simulink model "dampmaskine_rev9"  (R2017b)
settings: Solver=ode45  StartTime=0.0  StopTime=1000  RelTol=2e-6  EnableMultiTasking=on
values from neighbouring files (symbols this model uses):
  Bm = 2e-6    (= 2e-06)    [konstanter_rev9.m]
  CthV1 = 5    [konstanter_rev9.m]
  CthV2 = 50    [konstanter_rev9.m]
  Jm = Jmm + 0.5 * (0.015^2 * pi * 0.03 * jernMassefylde) * 0.015^2    (= 0.000106908078188)    [konstanter_rev9.m]
  Kd = stempelAreal*krumtapArm/2 * kd_ny * antalCylindre    (= 1.01787601976e-07)    [konstanter_rev9.m]
  kedelGodsVarmekapacitet = kedelOverflade*kedelGodsTykkelse * jernMassefylde * jernVarmefylde    (= 211.895159678)    [konstanter_rev9.m]
  kedelOverflade = 2 * (kedelDiameter / 2)^2 * pi + kedelDiameter * pi * kedelLength    (= 0.0403757487839)    [konstanter_rev9.m]
  kedelVandVarmekapacitet = kedelVolumen * vandMassefylde * vandVarmefylde    (= 2110.84160173)    [konstanter_rev9.m]
  kedelVolumen = (kedelDiameter / 2 - kedelGodsTykkelse)^2 * pi * (kedelLength - kedelGodsTykkelse*2)    (= 0.000504382700534)    [konstanter_rev9.m]
  Kp = 1/M    [Opgave33.m]    (also in konstanter_rev9.m = 3360.3; tfAfDamp_konstanter.m)
  Kvm = 1/(1-spild)*stempelAreal * slaglng / (2 * pi) * fyndningsgrad * antalCylindre    (= 9.25714285714e-07)    [konstanter_rev9.m]
  polPrRad = 13/(2*pi)    (= 2.06901426019)    [konstanter_rev9.m]
  RthV1 = 0.3    [konstanter_rev9.m]
  RthV2 = 0.1    [konstanter_rev9.m]
  startFriction = 0.005    [konstanter_rev9.m]
  tau_i = Ni/omega_c    (= 0.46511627907)    [Opgave33.m]    (also in konstanter_rev9.m = 32.05; tfAfDamp_konstanter.m = 32.0512820513)
  voltPerRad = voltPerRPM*60/2/pi    (= 0.019098593171)    [konstanter_rev9.m]
settings Model: Creator=chr  LastModifiedBy=tilfr
settings SolverCC: ZeroCrossAlgorithm=Adaptive
settings DataIOCC: MaxDataPoints=2000  SaveFinalState=on  SaveFormat=Array
settings OptimizationCC: ExpressionDepthLimit=2147483647  LifeSpan=inf
settings DebuggingCC: UnderspecifiedInitializationDetection=Classic  MergeDetectMultiDrivingBlocksExec=none  SolverPrmCheckMsg=warning  MultiTaskDSMMsg=warning  MultiTaskCondExecSysMsg=none  FcnCallInpInsideContextMsg=warning  StateNameClashWarn=warning  SFUnexpectedBacktrackingDiag=warning  SFNoUnconditionalDefaultTransitionDiag=warning  SFExecutionAtInitializationDiag=none
settings HardwareCC: ProdBitPerPointer=32  ProdBitPerSizeT=32  ProdBitPerPtrDiffT=32  ProdLargestAtomicFloat=None  ProdIntDivRoundTo=Undefined  ProdEndianess=Unspecified  ProdWordSize=32  ProdHWDeviceType=32-bit Generic
settings ModelReferenceCC: PropagateSignalLabelsOutOfModel=off
settings CodeAppCC: StateflowObjectComments=on
settings GRTTargetCC: TargetLangStandard=C89/C90 (ANSI)  GeneratePreprocessorConditionals=Disable all
settings ConfigComp: CovMetricSettings=dw  CovHtmlReporting=on  CovSaveCumulativeToWorkspaceVar=on  CovSaveSingleToWorkspaceVar=on  CovExternalEMLEnable=off
settings ConfigurationSet: Description=SimMechanics 2G

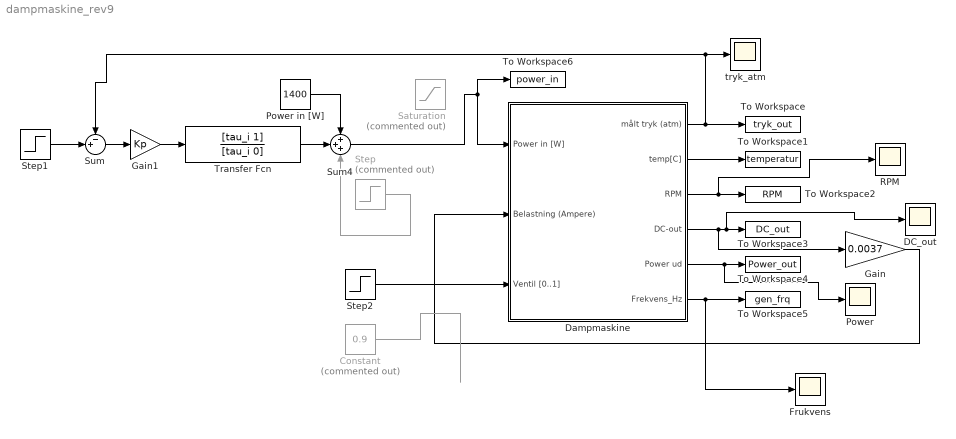
== system dampmaskine_rev9 ==
  Constant : Constant  Commented=on  Value=0.9
  DC_out : Scope
  Dampmaskine : Subsystem
  Frukvens : Scope
  Gain : Gain  Gain=0.0037
  Gain1 : Gain  Gain=Kp
  Power : Scope
  Power in [W] : Constant  Value=1400
  RPM : Scope
  Saturation : Saturate  Commented=on  UpperLimit=1400  LowerLimit=0
  Step : Step  Commented=on  Time=150  After=-50  SampleTime=0
  Step1 : Step  Time=0  After=3  SampleTime=0
  Step2 : Step  Time=500  Before=0.5  After=0.6  SampleTime=0
  Sum : Sum  Inputs=-+|
  Sum4 : Sum  Inputs=+++
  To Workspace : ToWorkspace  VariableName=tryk_out  SaveFormat=Timeseries  SampleTime=0.1
  To Workspace1 : ToWorkspace  VariableName=temperatur  SaveFormat=Timeseries  SampleTime=-1
  To Workspace2 : ToWorkspace  VariableName=RPM  SaveFormat=Timeseries  SampleTime=-1
  To Workspace3 : ToWorkspace  VariableName=DC_out  SaveFormat=Timeseries  SampleTime=-1
  To Workspace4 : ToWorkspace  VariableName=Power_out  SaveFormat=Timeseries  SampleTime=-1
  To Workspace5 : ToWorkspace  VariableName=gen_frq  SaveFormat=Timeseries  SampleTime=0.1
  To Workspace6 : ToWorkspace  VariableName=power_in  SaveFormat=Timeseries  SampleTime=0.1
  Transfer Fcn : TransferFcn  Numerator=[tau_i 1]  Denominator=[tau_i 0]
  tryk_atm : Scope
  wires:
  Step2/1 -> Dampmaskine/3(Ventil [0..1])
  Dampmaskine/3(RPM) -> RPM/1, To Workspace2/1
  Dampmaskine/6(Frekvens_Hz) -> Frukvens/1, To Workspace5/1
  Dampmaskine/5(Power ud) -> Power/1, To Workspace4/1
  Dampmaskine/2(temp[C]) -> To Workspace1/1
  Dampmaskine/4(DC-out) -> Gain/1, DC_out/1, To Workspace3/1
  Dampmaskine/1(målt tryk (atm)) -> Sum/1, tryk_atm/1, To Workspace/1
  Power in [W]/1 -> Sum4/1
  Step/1 -> Sum4/3
  Gain/1 -> Dampmaskine/2(Belastning (Ampere))
  Sum4/1 -> Dampmaskine/1(Power in [W]), To Workspace6/1
  Transfer Fcn/1 -> Sum4/2
  Gain1/1 -> Transfer Fcn/1
  Step1/1 -> Sum/2
  Sum/1 -> Gain1/1
  Constant/1 -> ?

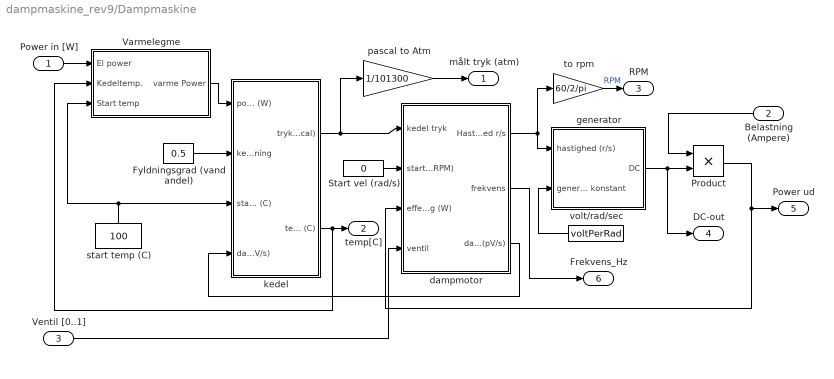
== system dampmaskine_rev9/Dampmaskine ==
  Power in [W] : Inport
  Belastning (Ampere) : Inport  Port=2
  Ventil [0..1] : Inport  Port=3
  Fyldningsgrad (vand andel) : Constant  Value=0.5
  Product : Product  RndMeth=Zero
  Start vel (rad/s) : Constant  Value=0
  Varmelegme : Subsystem
  dampmotor : Subsystem
  generator : Subsystem
  kedel : Subsystem
  pascal to Atm : Gain  Gain=1/101300
  start temp (C) : Constant  Value=100
  to rpm : Gain  Gain=60/2/pi
  volt/rad/sec : Constant  Value=voltPerRad
  målt tryk (atm) : Outport
  temp[C] : Outport  Port=2
  RPM : Outport  Port=3
  DC-out : Outport  Port=4
  Power ud : Outport  Port=5
  Frekvens_Hz : Outport  Port=6
  wires:
  Fyldningsgrad (vand andel)/1 -> kedel/2(kedel fyldning)
  start temp (C)/1 -> Varmelegme/3(Start temp), kedel/3(start temp (C))
  dampmotor/1(Hastighed r/s) -> generator/1(hastighed (r/s)), to rpm/1
  volt/rad/sec/1 -> generator/2(generator konstant)
  pascal to Atm/1 -> målt tryk (atm)/1
  Start vel (rad/s)/1 -> dampmotor/2(start vel (RPM))
  kedel/1(tryk (pascal)) -> pascal to Atm/1, dampmotor/1(kedel tryk)
  to rpm/1 -> RPM/1  "RPM"
  kedel/2(temp (C)) -> Varmelegme/2(Kedeltemp.), temp[C]/1
  dampmotor/3(damp forbrug (pV/s)) -> kedel/4(dampflow (pV/s))
  Belastning (Ampere)/1 -> Product/1
  generator/1(DC) -> Product/2, DC-out/1
  Product/1 -> dampmotor/3(effekt forbrug (W)), Power ud/1
  Power in [W]/1 -> Varmelegme/1(El power)
  Varmelegme/1(varme Power) -> kedel/1(power ind  (W))
  Ventil [0..1]/1 -> dampmotor/4(ventil)
  dampmotor/2(frekvens) -> Frekvens_Hz/1

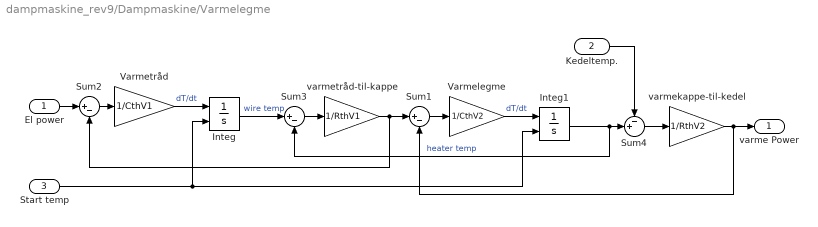
== system dampmaskine_rev9/Dampmaskine/Varmelegme ==
  El power : Inport
  Kedeltemp. : Inport  Port=2
  Start temp : Inport  Port=3
  Integ : Integrator  InitialConditionSource=external
  Integ1 : Integrator  InitialConditionSource=external
  Sum1 : Sum  Inputs=|+-
  Sum2 : Sum  Inputs=|+-
  Sum3 : Sum  Inputs=|+-
  Sum4 : Sum  Inputs=-+|
  Varmelegme : Gain  Gain=1/CthV2
  Varmetråd : Gain  Gain=1/CthV1
  varmekappe-til-kedel : Gain  Gain=1/RthV2
  varmetråd-til-kappe : Gain  Gain=1/RthV1
  varme Power : Outport
  wires:
  Sum3/1 -> varmetråd-til-kappe/1
  El power/1 -> Sum2/1
  Varmetråd/1 -> Integ/1  "dT/dt"
  Sum2/1 -> Varmetråd/1
  Integ/1 -> Sum3/1  "wire temp"
  Sum4/1 -> varmekappe-til-kedel/1
  Kedeltemp./1 -> Sum4/1
  varmetråd-til-kappe/1 -> Sum1/1, Sum2/2
  Varmelegme/1 -> Integ1/1  "dT/dt"
  Sum1/1 -> Varmelegme/1
  Integ1/1 -> Sum4/2, Sum3/2  "heater temp"
  varmekappe-til-kedel/1 -> varme Power/1, Sum1/2
  Start temp/1 -> Integ1/2, Integ/2

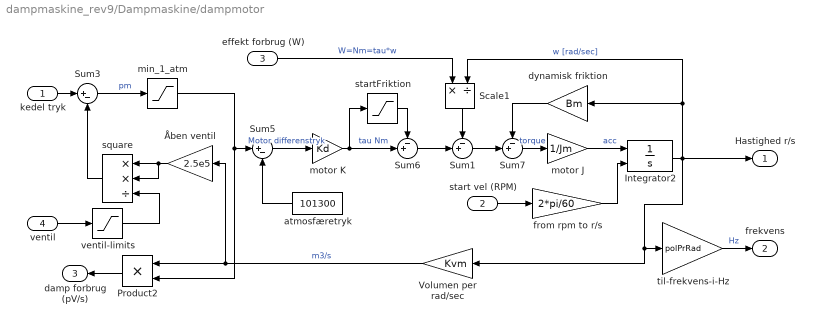
== system dampmaskine_rev9/Dampmaskine/dampmotor ==
  kedel tryk : Inport
  start vel (RPM) : Inport  Port=2
  effekt forbrug (W) : Inport  Port=3
  ventil : Inport  Port=4
  Integrator2 : Integrator  InitialConditionSource=external  InitialCondition=1332/60*2*pi  LimitOutput=on  LowerSaturationLimit=0.001
  Product2 : Product  RndMeth=Zero
  Scale1 : Product  Inputs=*/
  Sum1 : Sum  Inputs=-+|
  Sum3 : Sum  Inputs=|+-
  Sum5 : Sum  Inputs=|+-
  Sum6 : Sum  Inputs=-+|
  Sum7 : Sum  Inputs=-+|
  Volumen per rad/sec : Gain  Gain=Kvm
  atmosfæretryk : Constant  Value=101300
  dynamisk friktion : Gain  Gain=Bm
  from rpm to r/s : Gain  Gain=2*pi/60
  min_1_atm : Saturate  UpperLimit=1e8  LowerLimit=101300
  motor J : Gain  Gain=1/Jm
  motor K : Gain  Gain=Kd
  square : Product  Inputs=**/  RndMeth=Zero
  startFriktion : Saturate  UpperLimit=startFriction  LowerLimit=-startFriction
  til-frekvens-i-Hz : Gain  Gain=polPrRad
  ventil-limits : Saturate  UpperLimit=1  LowerLimit=1e-5
  Åben ventil : Gain  Gain=2.5e5
  Hastighed r/s : Outport
  frekvens : Outport  Port=2
  damp forbrug (pV/s) : Outport  Port=3
  wires:
  Sum5/1 -> motor K/1  "Motor differenstryk"
  atmosfæretryk/1 -> Sum5/2
  Sum7/1 -> motor J/1  "torque"
  motor J/1 -> Integrator2/1  "acc"
  Integrator2/1 -> Hastighed r/s/1, Scale1/2, dynamisk friktion/1, Volumen per rad/sec/1, til-frekvens-i-Hz/1  "w [rad/sec]"
  dynamisk friktion/1 -> Sum7/1
  motor K/1 -> startFriktion/1, Sum6/2  "tau Nm"
  Sum3/1 -> min_1_atm/1  "pm"
  Åben ventil/1 -> square/2, square/1
  Volumen per rad/sec/1 -> Åben ventil/1, Product2/1  "m3/s"
  min_1_atm/1 -> Product2/2, Sum5/1
  kedel tryk/1 -> Sum3/1
  Product2/1 -> damp forbrug (pV/s)/1
  effekt forbrug (W)/1 -> Scale1/1  "W=Nm=tau*w"
  square/1 -> Sum3/2
  start vel (RPM)/1 -> from rpm to r/s/1
  from rpm to r/s/1 -> Integrator2/2
  ventil/1 -> ventil-limits/1
  ventil-limits/1 -> square/3
  til-frekvens-i-Hz/1 -> frekvens/1  "Hz"
  Sum1/1 -> Sum7/2
  Sum6/1 -> Sum1/2
  Scale1/1 -> Sum1/1
  startFriktion/1 -> Sum6/1

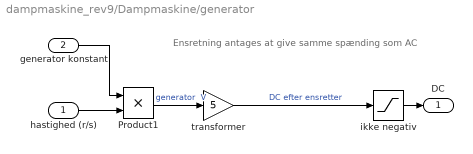
== system dampmaskine_rev9/Dampmaskine/generator ==
  note: Ensretning antages at give samme spænding som AC
  hastighed (r/s) : Inport
  generator konstant : Inport  Port=2
  Product1 : Product  RndMeth=Zero
  ikke negativ : Saturate  UpperLimit=300  LowerLimit=0
  transformer : Gain  Gain=5
  DC : Outport
  wires:
  hastighed (r/s)/1 -> Product1/2
  Product1/1 -> transformer/1  "generator  V"
  generator konstant/1 -> Product1/1
  transformer/1 -> ikke negativ/1  "DC efter ensretter"
  ikke negativ/1 -> DC/1

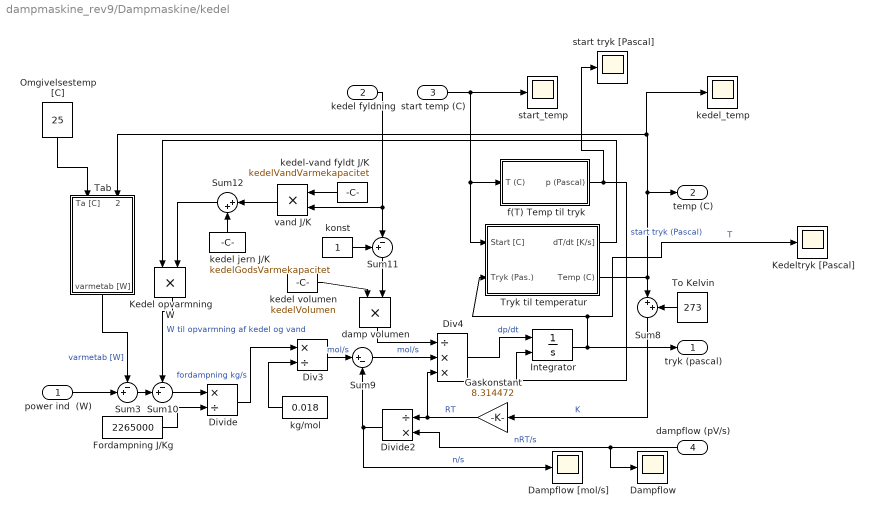
== system dampmaskine_rev9/Dampmaskine/kedel ==
  power ind  (W) : Inport
  kedel fyldning : Inport  Port=2
  start temp (C) : Inport  Port=3
  dampflow (pV/s) : Inport  Port=4
  Dampflow : Scope
  Dampflow [mol/s] : Scope
  Div3 : Product  Inputs=*/
  Div4 : Product  Inputs=/**
  Divide : Product  Inputs=*/
  Divide2 : Product  Inputs=/*
  Fordampning J/Kg : Constant  Value=2265000
  Gaskonstant : Gain  Gain=8.314472
  Integrator : Integrator  InitialConditionSource=external  InitialCondition=122.7
  Kedel opvarmning W : Product  RndMeth=Zero
  Kedeltryk [Pascal] : Scope
  Omgivelsestemp [C] : Constant  Value=25
  Sum10 : Sum  Inputs=-+|
  Sum11 : Sum  Inputs=+-|
  Sum12 : Sum  Inputs=|++
  Sum3 : Sum  Inputs=-+|
  Sum8 : Sum  Inputs=|++
  Sum9 : Sum  Inputs=|+-
  Tab : Subsystem
  To Kelvin : Constant  Value=273
  Tryk til temperatur : Subsystem
  damp volumen : Product  RndMeth=Zero
  f(T) Temp til tryk : Subsystem
  kedel jern J/K : Constant  Value=kedelGodsVarmekapacitet
  "kedel volumen " : Constant  Value=kedelVolumen
  kedel-vand fyldt J/K : Constant  Value=kedelVandVarmekapacitet
  kedel_temp : Scope
  kg/mol : Constant  Value=0.018
  konst : Constant
  start tryk [Pascal] : Scope
  "start_temp " : Scope
  vand J/K : Product  RndMeth=Zero
  tryk (pascal) : Outport
  temp (C) : Outport  Port=2
  wires:
  f(T) Temp til tryk/1(p (Pascal)) -> start tryk [Pascal]/1, Integrator/2  "start tryk (Pascal)"
  Gaskonstant/1 -> Div4/3, Divide2/1  "RT"
  Divide2/1 -> Dampflow [mol/s]/1, Sum9/2  "n/s"
  dampflow (pV/s)/1 -> Dampflow/1, Divide2/2  "nRT/s"
  Fordampning J/Kg/1 -> Divide/2
  Divide/1 -> Div3/1  "fordampning kg/s"
  kg/mol/1 -> Div3/2
  Div3/1 -> Sum9/1  "mol/s"
  Integrator/1 -> tryk (pascal)/1, Kedeltryk [Pascal]/1, Tryk til temperatur/2(Tryk (Pas.))  "T"
  Div4/1 -> Integrator/1  "dp/dt"
  To Kelvin/1 -> Sum8/2
  Sum8/1 -> Gaskonstant/1  "K"
  Sum3/1 -> Sum10/2
  Kedel opvarmning W/1 -> Sum10/1  "W til opvarmning af kedel og vand"
  Sum10/1 -> Divide/1
  Sum9/1 -> Div4/2  "mol/s"
  damp volumen/1 -> Div4/1
  "kedel volumen "/1 -> damp volumen/1
  Sum11/1 -> damp volumen/2
  kedel fyldning/1 -> Sum11/2, vand J/K/2
  kedel-vand fyldt J/K/1 -> vand J/K/1
  vand J/K/1 -> Sum12/1
  Sum12/1 -> Kedel opvarmning W/2
  kedel jern J/K/1 -> Sum12/2
  konst/1 -> Sum11/1
  start temp (C)/1 -> Tryk til temperatur/1(Start [C]), f(T) Temp til tryk/1(T (C)), "start_temp "/1
  Tryk til temperatur/2(Temp (C)) -> kedel_temp/1, Tab/2(Kedel temp), temp (C)/1, Sum8/1
  Tryk til temperatur/1(" dT/dt [K/s]") -> Kedel opvarmning W/1
  Tab/1(varmetab [W]) -> Sum3/1  "varmetab [W]"
  Omgivelsestemp [C]/1 -> Tab/1(Ta [C])
  power ind  (W)/1 -> Sum3/2

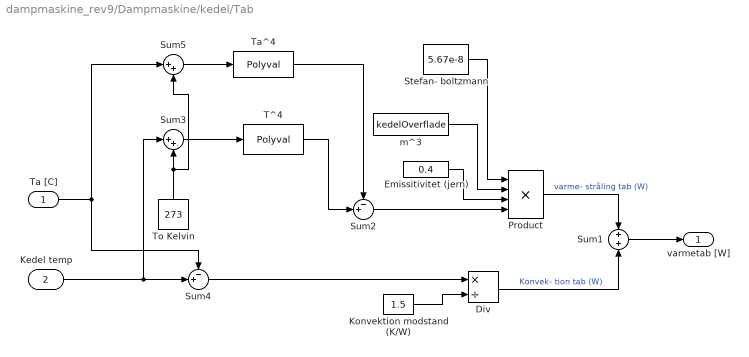
== system dampmaskine_rev9/Dampmaskine/kedel/Tab ==
  Ta [C] : Inport
  Kedel temp : Inport  Port=2
  Div : Product  Inputs=*/
  Emissitivitet (jern) : Constant  Value=0.4
  Konvektion modstand (K/W) : Constant  Value=1.5
  Product : Product  Inputs=4  RndMeth=Zero
  Stefan- boltzmann : Constant  Value=5.67e-8
  Sum1 : Sum  Inputs=+|+
  Sum2 : Sum  Inputs=-+|
  Sum3 : Sum  Inputs=|++
  Sum4 : Sum  Inputs=-+|
  Sum5 : Sum  Inputs=|++
  T^4 : Polyval  Coefs=[1,0,0,0,0 ]
  Ta^4 : Polyval  Coefs=[1,0,0,0,0 ]
  To Kelvin : Constant  Value=273
  m^3 : Constant  Value=kedelOverflade
  varmetab [W] : Outport
  wires:
  Ta^4/1 -> Sum2/1
  Kedel temp/1 -> Sum3/1, Sum4/2
  Sum2/1 -> Product/4
  Ta [C]/1 -> Sum4/1, Sum5/1
  Stefan- boltzmann/1 -> Product/1
  Emissitivitet (jern)/1 -> Product/3
  Sum3/1 -> T^4/1
  T^4/1 -> Sum2/2
  Sum4/1 -> Div/1
  Sum5/1 -> Ta^4/1
  Div/1 -> Sum1/2  "Konvek- tion tab (W)"
  Konvektion modstand (K/W)/1 -> Div/2
  m^3/1 -> Product/2
  Product/1 -> Sum1/1  "varme- stråling tab (W)"
  Sum1/1 -> varmetab [W]/1
  To Kelvin/1 -> Sum5/2, Sum3/2

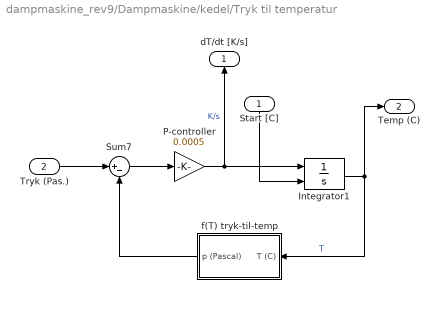
== system dampmaskine_rev9/Dampmaskine/kedel/Tryk til temperatur ==
  Start [C] : Inport
  Tryk (Pas.) : Inport  Port=2
  Integrator1 : Integrator  InitialConditionSource=external  InitialCondition=122.7
  "P-controller " : Gain  Gain=0.0005
  Sum7 : Sum  Inputs=|+-
  f(T) tryk-til-temp : Subsystem
  " dT/dt [K/s]" : Outport
  Temp (C) : Outport  Port=2
  wires:
  Sum7/1 -> "P-controller "/1
  Start [C]/1 -> Integrator1/2
  f(T) tryk-til-temp/1(p (Pascal)) -> Sum7/2
  "P-controller "/1 -> " dT/dt [K/s]"/1, Integrator1/1  "K/s"
  Tryk (Pas.)/1 -> Sum7/1
  Integrator1/1 -> Temp (C)/1, f(T) tryk-til-temp/1(T (C))  "T"

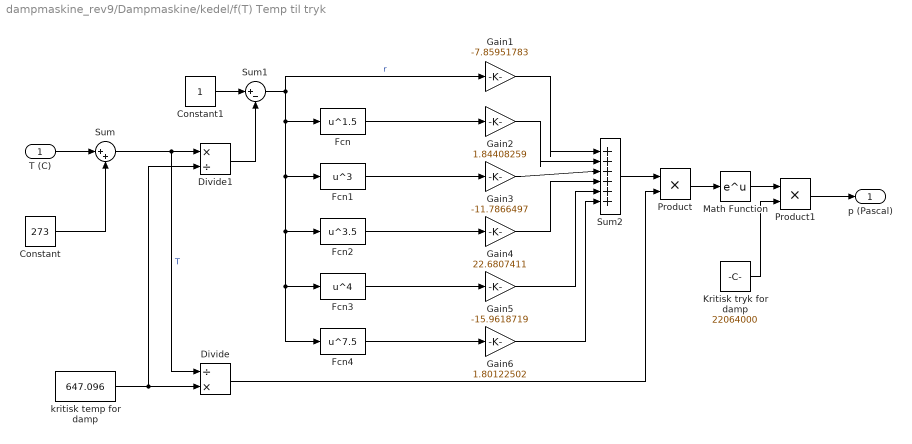
== system dampmaskine_rev9/Dampmaskine/kedel/f(T) Temp til tryk ==
  T (C) : Inport
  Constant : Constant  Value=273
  Constant1 : Constant
  Divide : Product  Inputs=/*
  Divide1 : Product  Inputs=*/
  Fcn : Fcn  Expr=u^1.5
  Fcn1 : Fcn  Expr=u^3
  Fcn2 : Fcn  Expr=u^3.5
  Fcn3 : Fcn  Expr=u^4
  Fcn4 : Fcn  Expr=u^7.5
  Gain1 : Gain  Gain=-7.85951783
  Gain2 : Gain  Gain=1.84408259
  Gain3 : Gain  Gain=-11.7866497
  Gain4 : Gain  Gain=22.6807411
  Gain5 : Gain  Gain=-15.9618719
  Gain6 : Gain  Gain=1.80122502
  Kritisk tryk for damp : Constant  Value=22064000
  Math Function : Math  SaturateOnIntegerOverflow=on
  Product : Product  RndMeth=Zero
  Product1 : Product  RndMeth=Zero
  Sum : Sum  Inputs=|++
  Sum1 : Sum  Inputs=|+-
  Sum2 : Sum  Inputs=|++++++
  kritisk temp for damp : Constant  Value=647.096
  p (Pascal) : Outport
  wires:
  Fcn2/1 -> Gain4/1
  Fcn4/1 -> Gain6/1
  Fcn3/1 -> Gain5/1
  Fcn1/1 -> Gain3/1
  Fcn/1 -> Gain2/1
  Product1/1 -> p (Pascal)/1
  Math Function/1 -> Product1/1
  Kritisk tryk for damp/1 -> Product1/2
  Product/1 -> Math Function/1
  Divide/1 -> Product/2
  Sum2/1 -> Product/1
  Gain5/1 -> Sum2/5
  Gain6/1 -> Sum2/6
  Gain4/1 -> Sum2/4
  Gain3/1 -> Sum2/3
  Gain2/1 -> Sum2/2
  Gain1/1 -> Sum2/1
  kritisk temp for damp/1 -> Divide/2, Divide1/2
  Sum1/1 -> Fcn2/1, Fcn4/1, Fcn3/1, Fcn1/1, Fcn/1, Gain1/1  "r"
  Sum/1 -> Divide/1, Divide1/1  "T"
  Constant1/1 -> Sum1/1
  Divide1/1 -> Sum1/2
  Constant/1 -> Sum/2
  T (C)/1 -> Sum/1

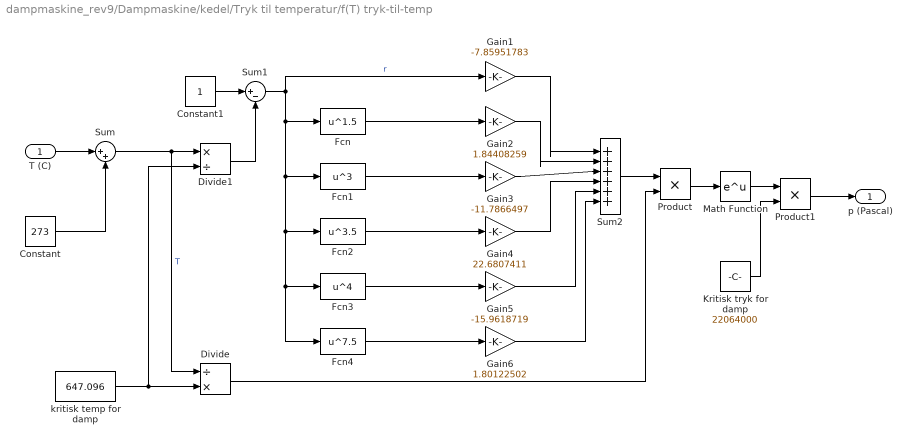
== system dampmaskine_rev9/Dampmaskine/kedel/Tryk til temperatur/f(T) tryk-til-temp ==
  T (C) : Inport
  Constant : Constant  Value=273
  Constant1 : Constant
  Divide : Product  Inputs=/*
  Divide1 : Product  Inputs=*/
  Fcn : Fcn  Expr=u^1.5
  Fcn1 : Fcn  Expr=u^3
  Fcn2 : Fcn  Expr=u^3.5
  Fcn3 : Fcn  Expr=u^4
  Fcn4 : Fcn  Expr=u^7.5
  Gain1 : Gain  Gain=-7.85951783
  Gain2 : Gain  Gain=1.84408259
  Gain3 : Gain  Gain=-11.7866497
  Gain4 : Gain  Gain=22.6807411
  Gain5 : Gain  Gain=-15.9618719
  Gain6 : Gain  Gain=1.80122502
  Kritisk tryk for damp : Constant  Value=22064000
  Math Function : Math  SaturateOnIntegerOverflow=on
  Product : Product  RndMeth=Zero
  Product1 : Product  RndMeth=Zero
  Sum : Sum  Inputs=|++
  Sum1 : Sum  Inputs=|+-
  Sum2 : Sum  Inputs=|++++++
  kritisk temp for damp : Constant  Value=647.096
  p (Pascal) : Outport
  wires:
  T (C)/1 -> Sum/1
  Constant/1 -> Sum/2
  Divide1/1 -> Sum1/2
  Constant1/1 -> Sum1/1
  Sum/1 -> Divide1/1, Divide/1  "T"
  Sum1/1 -> Gain1/1, Fcn/1, Fcn1/1, Fcn3/1, Fcn4/1, Fcn2/1  "r"
  kritisk temp for damp/1 -> Divide1/2, Divide/2
  Gain1/1 -> Sum2/1
  Gain2/1 -> Sum2/2
  Gain3/1 -> Sum2/3
  Gain4/1 -> Sum2/4
  Gain6/1 -> Sum2/6
  Gain5/1 -> Sum2/5
  Sum2/1 -> Product/1
  Divide/1 -> Product/2
  Product/1 -> Math Function/1
  Kritisk tryk for damp/1 -> Product1/2
  Math Function/1 -> Product1/1
  Product1/1 -> p (Pascal)/1
  Fcn/1 -> Gain2/1
  Fcn1/1 -> Gain3/1
  Fcn3/1 -> Gain5/1
  Fcn4/1 -> Gain6/1
  Fcn2/1 -> Gain4/1
